simulink subsystem "TankLevelDynamics_SimplifiedNonlinear_Simulink"  (R2020b)
settings: Solver=VariableStepAuto  StartTime=0.0  StopTime=10.0  RelTol=1e-3
undefined symbols (not defined in the file): a_r, a_s, gamma, h, k_vv, x_r_e, x_s_e
settings Model: Creator=Jonas  LastModifiedBy=Jonas

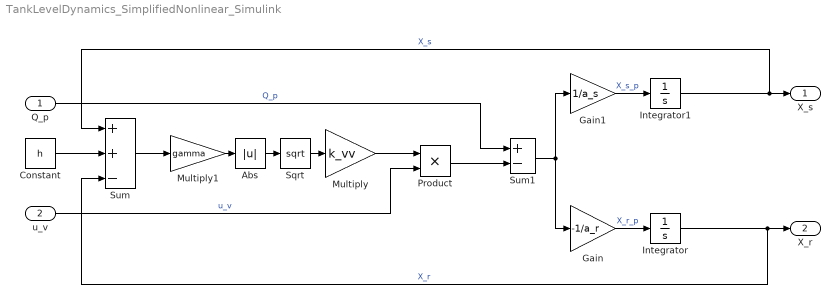
== system TankLevelDynamics_SimplifiedNonlinear_Simulink ==
  Q_p : Inport
  u_v : Inport  Port=2
  Abs : Abs
  Constant : Constant  Value=h
  Gain : Gain  Gain=-1/a_r
  Gain1 : Gain  Gain=1/a_s
  Integrator : Integrator  InitialCondition=x_s_e
  Integrator1 : Integrator  InitialCondition=x_r_e
  Multiply : Gain  Gain=k_vv
  Multiply1 : Gain  Gain=gamma
  Product : Product
  Sqrt : Sqrt  SaturateOnIntegerOverflow=on
  Sum : Sum  Inputs=++-
  Sum1 : Sum  Inputs=+-
  X_s : Outport
  X_r : Outport  Port=2
  wires:
  Multiply/1 -> Product/1
  Product/1 -> Sum1/2
  Gain1/1 -> Integrator1/1  "X_s_p"
  Abs/1 -> Sqrt/1
  Sqrt/1 -> Multiply/1
  Constant/1 -> Sum/2
  Sum/1 -> Multiply1/1
  Integrator1/1 -> Sum/1, X_s/1  "X_s"
  u_v/1 -> Product/2  "u_v"
  Gain/1 -> Integrator/1  "X_r_p"
  Integrator/1 -> Sum/3, X_r/1  "X_r"
  Multiply1/1 -> Abs/1
  Q_p/1 -> Sum1/1  "Q_p"
  Sum1/1 -> Gain/1, Gain1/1
